simulink model "Left_Ventricular_PV_Loop_Control_2017b"  (R2017b)
settings: Solver=ode14x  StartTime=0.0  StopTime=Sim_Time  FixedStep=1/1024  MaxStep=0.01  MinStep=1E-6  RelTol=1e-5
values from neighbouring files (symbols this model uses):
  Force_Rate = 500    [Left_Ventricular_PV_Loop_Variable_Load_and_Plot.m]
  Iso_Contraction_Offset = 1    [Left_Ventricular_PV_Loop_Variable_Load_and_Plot.m]
  Resistance = 0.045    [Left_Ventricular_PV_Loop_Variable_Load_and_Plot.m]
  Systolic_Ejection_Increase = 9    [Left_Ventricular_PV_Loop_Variable_Load_and_Plot.m]
  Systolic_Ejection_Offset = [20 20]    [Left_Ventricular_PV_Loop_Variable_Load_and_Plot.m]
  Variable_Ea_C0 = [235.76 235.76 235.76 220.7 205.63 190.56 175.5 160.43]    [Left_Ventricular_PV_Loop_Variable_Load_and_Plot.m]
  Variable_Ea_C1 = [-1.4054 -1.4054 -1.4054 -1.3994 -1.3934 -1.3874 -1.3814 -1.3754]    [Left_Ventricular_PV_Loop_Variable_Load_and_Plot.m]
  Variable_EDPVR_B0 = -0.010234    [Left_Ventricular_PV_Loop_Variable_Load_and_Plot.m]
  Variable_EDPVR_B1 = 0.15836    [Left_Ventricular_PV_Loop_Variable_Load_and_Plot.m]
  Variable_EDPVR_B2 = -0.0025351    [Left_Ventricular_PV_Loop_Variable_Load_and_Plot.m]
  Variable_EDPVR_B3 = 1.4046E-5    (= 1.4046e-05)    [Left_Ventricular_PV_Loop_Variable_Load_and_Plot.m]
  Variable_ESPVR_A0 = 72.586    [Left_Ventricular_PV_Loop_Variable_Load_and_Plot.m]
  Variable_ESPVR_A1 = [0.99741 0.99741]    [Left_Ventricular_PV_Loop_Variable_Load_and_Plot.m]
libraries: fl_lib x15, nesl_utility x9, sh_lib x4, simulink x3
settings Model: SimulationMode=accelerator  Creator=ULCajunAdmin  LastModifiedBy=jmk9354
settings SolverCC: ExtrapolationOrder=2  MaxConsecutiveMinStep=5  ZeroCrossAlgorithm=Adaptive  SolverResetMethod=Robust
settings DataIOCC: SaveFormat=StructureWithTime
settings OptimizationCC: LifeSpan=inf
settings DebuggingCC: IgnoredZcDiagnostic=none  SFUnexpectedBacktrackingDiag=warning  SFNoUnconditionalDefaultTransitionDiag=warning  SFExecutionAtInitializationDiag=none
settings HardwareCC: ProdBitPerPointer=32  ProdBitPerSizeT=32  ProdBitPerPtrDiffT=32  ProdLargestAtomicFloat=None  ProdIntDivRoundTo=Undefined  ProdEndianess=Unspecified  ProdWordSize=32  ProdHWDeviceType=32-bit Generic
settings ModelReferenceCC: PropagateSignalLabelsOutOfModel=off
settings CodeAppCC: StateflowObjectComments=on
settings GRTTargetCC: TargetLangStandard=C89/C90 (ANSI)  GeneratePreprocessorConditionals=Disable all
settings ConfigComp: CovMetricSettings=dw  CovHtmlReporting=on  CovSaveCumulativeToWorkspaceVar=on  CovSaveSingleToWorkspaceVar=on  CovExternalEMLEnable=off
settings SimscapeCC: SimscapeNormalizeSystem=off

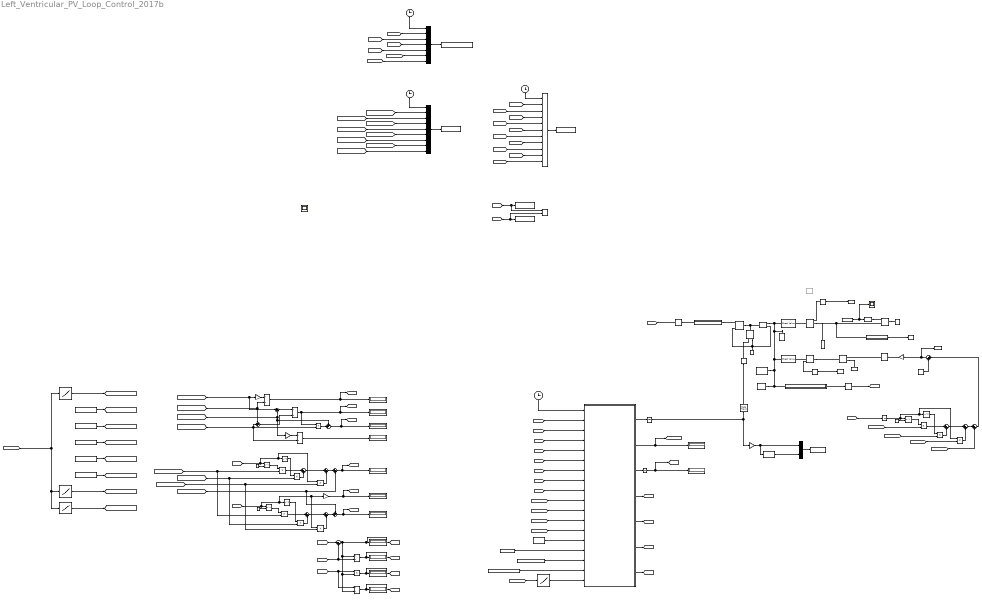
== system Left_Ventricular_PV_Loop_Control_2017b ==
   {,,,} (4 alike) : Product
  " " : Constant  Value=3
   {,,,,} (5 alike) : Product  Inputs=*/
  " " : Constant  Value=3
  " " : Constant  Value=3
  " " : Product  Inputs=**
  " " : Product  Inputs=**
  "            " : Gain  Gain=-1
  "                             " : Gain  Gain=-1
  "                                              " : Product
  "                                                              " : Product
  "                                                               " : Gain
  "                                                                        " : Product
  "                                                                            " : Product
  "                                                                            1" : Product
  Aortic Pressure Sensor : Subsystem
  Bus Creator : BusCreator  Inputs=9
  Bus Creator1 : BusCreator  Inputs=11
  Bus Creator2 : BusCreator  Inputs=2
  Bus Creator3 : BusCreator  Inputs=7
  Check Valve (Aortic Valve) Max Passage Area: 3.14*0.46^2 Cracking Pressure: 0.01 psi = 0.5 mmHg Max Opening Pressure: 0.02 psi = 1 mmHg : sh_lib/Valves/Directional Valves/Check Valve  area_max=3.14*0.46^2 in^2  pres_crack=0.01 psi  pres_max=0.02 psi  C_d=0.7  A_leak=1e-12 m^2  lam_spec=2  B_lam=0.999  Re_cr=12  dynamic=0  tau=0.001 s  area_init=1e-12 m^2
      settings: SourceProductName=Simscape Fluids  SourceProductBaseCode=SH
  "Check Valve (Mitral Valve) Max Passage Area: 3.14*0.46^2 Cracking Pressure: 0.01 psi = 0.5 mmHg Max Opening Pressure: 0.02 psi = 1 mmHg " : sh_lib/Valves/Directional Valves/Check Valve  area_max=3.14*0.46^2 in^2  pres_crack=0.01 psi  pres_max=0.02 psi  C_d=0.7  A_leak=1e-12 m^2  lam_spec=2  B_lam=0.999  Re_cr=12  dynamic=0  tau=0.001 s  area_init=1e-12 m^2
      settings: SourceProductName=Simscape Fluids  SourceProductBaseCode=SH
  Clock{,1..3} (4 alike) : Clock
  Constant Volume Hydraulic Chamber Chamber internal Diameter: 2 inch Cylindrical chamber length: 3 inch : fl_lib/Hydraulic/Hydraulic Elements/Constant Volume Hydraulic Chamber  ch_sp=2  wall_type=1  ch_volume=200 cm^3  d_in=2 in  length=3 in  pr_r_coef=1.2e-12 m/Pa  time_const=0.01 s  k_sh=1.4  pressure_specify=off  pressure_priority=High  pressure=0 Pa  pressure_nominal_specify=off  pressure_nominal_unit=Pa  pressure_nominal_value=1  diameter_incr_specify=off  diameter_incr_priority=High  diameter_incr=2 in  diameter_incr_nominal_specify=off  diameter_incr_nominal_unit=m  diameter_incr_nominal_value=1  flow_rate_specify=off  flow_rate_priority=None  flow_rate=0.001 m^3/s  flow_rate_nominal_specify=off  flow_rate_nominal_unit=m^3/s  flow_rate_nominal_value=1
      settings: SourceProductName=Simscape  SourceProductBaseCode=SS
  Cubic : Math  Operator=pow  SaturateOnIntegerOverflow=on
  "Cubic " : Math  Operator=pow  SaturateOnIntegerOverflow=on
  "Cubic " : Math  Operator=pow  SaturateOnIntegerOverflow=on
  "Discrete Derivative " : simulink/Discrete/Discrete Derivative  gainval=1.0  ICPrevScaledInput=0.0  OutMin=[]  OutMax=[]  OutDataType=fixdt(1, 16)  OutScaling=2^-10  DoSatur=off
  "EDPVR - B0 " : Constant  Value=Variable_EDPVR_B0  SampleTime=1/1024
  "EDPVR - B1 " : Constant  Value=Variable_EDPVR_B1  SampleTime=1/1024
  "EDPVR - B2 " : Constant  Value=Variable_EDPVR_B2  SampleTime=1/1024
  "EDPVR - B3 " : Constant  Value=Variable_EDPVR_B3  SampleTime=1/1024
  "ESPVR - A0 " : Constant  Value=Variable_ESPVR_A0  SampleTime=1/1024
  ESPVR - A1 1-D Lookup Table : Lookup_n-D  NumberOfTableDimensions=1  BreakpointsSpecification=Even spacing  BreakpointsForDimension1=[-5:5]  Table=Variable_ESPVR_A1  InterpMethod=Nearest  ExtrapMethod=Clip  UseLastTableValue=on  InternalRulePriority=Speed  RndMeth=Simplest  InputSameDT=on
  Ea - C0 1-D Lookup Table : Lookup_n-D  NumberOfTableDimensions=1  BreakpointsSpecification=Even spacing  BreakpointsForDimension1=[-5:5]  Table=Variable_Ea_C0  InterpMethod=Nearest  ExtrapMethod=Clip  UseLastTableValue=on  InternalRulePriority=Speed  RndMeth=Simplest  InputSameDT=on
  Ea - C1 1-D Lookup Table : Lookup_n-D  NumberOfTableDimensions=1  BreakpointsSpecification=Even spacing  BreakpointsForDimension1=[-5:5]  Table=Variable_Ea_C1  InterpMethod=Nearest  ExtrapMethod=Clip  UseLastTableValue=on  InternalRulePriority=Speed  RndMeth=Simplest  InputSameDT=on
  Force Rate : Constant  Value=Force_Rate  SampleTime=1/1024
  Gain2 : Gain  Gain=-1
  Heart Beat Cycle Number : Display
  Heart Rate : Display
  Hydraulic Flow Rate Sensor : fl_lib/Hydraulic/Hydraulic Sensors/Hydraulic Flow Rate Sensor
      settings: SourceProductName=Simscape
  "Hydraulic Flow Rate Sensor " : fl_lib/Hydraulic/Hydraulic Sensors/Hydraulic Flow Rate Sensor
      settings: SourceProductName=Simscape
  Hydraulic Fluid Glycerol/Water Mixture : fl_lib/Hydraulic/Hydraulic Utilities/Custom Hydraulic Fluid  density=1107.1 kg/m^3  viscosity_kin=3.3 cSt  bulk=0.8e9 Pa  alpha=0.005  range_error=2
      settings: SourceProductName=Simscape  SourceProductBaseCode=SS
  "Hydraulic Pressure Source " : fl_lib/Hydraulic/Hydraulic Sources/Hydraulic Pressure Source
      settings: SourceProductName=Simscape  SourceProductBaseCode=SS
  "Hydraulic Reference " : fl_lib/Hydraulic/Hydraulic Elements/Hydraulic Reference
      settings: SourceProductName=Simscape
  "Hydraulic Reference   " : fl_lib/Hydraulic/Hydraulic Elements/Hydraulic Reference
      settings: SourceProductName=Simscape
  "Ideal Force Source " : fl_lib/Mechanical/Mechanical Sources/Ideal Force Source
  "Ideal Translational Motion Sensor Initial Position: 0 inch " : fl_lib/Mechanical/Mechanical Sensors/Ideal Translational Motion Sensor  offset=0 in
  Isovolumetric Contraction Offset : Constant  Value=Iso_Contraction_Offset  SampleTime=1/1024
  LAP [mmHg] Offset : Constant  Value=2
  Left Ventricle Pressure Sensor : Subsystem
  Left Ventricular Arterial Elastance [mmHg/mL] : Display
  Left Ventricular Ejection Fraction : Display
  Left Ventricular End-Diastolic Pressure [mmHg] : Display
  Left Ventricular End-Diastolic Volume [mL] : Display
  Left Ventricular End-Isovolumetric Relaxation Pressure [mmHg] : Display
  Left Ventricular End-Isovolumetric Relaxation Volume [mL] : Display
  Left Ventricular End-Systolic Pressure [mmHg] : Display
  Left Ventricular End-Systolic Volume [mL] : Display
  Left Ventricular Stroke Volume [mL] : Display
  Left Ventricular Stroke Work [mmHg*mL] : Display
  Left Ventricular Volume Conversion : Subsystem
  Mechanical Translational Reference : fl_lib/Mechanical/Translational Elements/Mechanical Translational Reference
  "Needle Valve Orifice Diameter: 0.5 inch Needle Cone Angle: 90 degrees " : sh_lib/Valves/Flow Control Valves/Needle Valve  d_orif=0.5 in  cone_angle=90 deg  x_0=0 in  C_d=0.65  A_leak=1e-12 m^2  lam_spec=2  B_lam=0.999  Re_cr=10
      settings: SourceProductName=Simscape Fluids  SourceProductBaseCode=SH
  Needle Valve Resistance: Variable : Constant  Value=Resistance  VectorParams1D=off
  PS-Simulink Converter (mL/min) : nesl_utility/PS-Simulink Converter  PhysicalDomain=network_engine_domain  SubClassName=ps_output  LeftPortType=input  RightPortType=output  PseudoPeriodic=off  Frequencies=[]  Unit=cm^3/min  AffineConversion=off
  "PS-Simulink Converter (mL/min) " : nesl_utility/PS-Simulink Converter  PhysicalDomain=network_engine_domain  SubClassName=ps_output  LeftPortType=input  RightPortType=output  PseudoPeriodic=off  Frequencies=[]  Unit=cm^3/min  AffineConversion=off
  Piston Cross-Sectional Area : Constant  Value=pi*2.54^2  SampleTime=1/1024
  Ramp : simulink/Sources/Ramp  Commented=on  slope=0.0125  start=2  X0=0
  Rate Transition 512 Hz : RateTransition  OutPortSampleTime=1/512
  Rate Transition to 512 Hz : RateTransition  OutPortSampleTime=1/512
  "Rate Transition to 512 Hz " : RateTransition  OutPortSampleTime=1/512
  Scope3 : Scope
  "Simulink-PS Converter (Newtons) " : nesl_utility/Simulink-PS Converter  PhysicalDomain=network_engine_domain  SubClassName=ps_input  LeftPortType=input  RightPortType=output  PseudoPeriodic=off  Frequencies=[]  NoiseDistribution=none  NoiseParameters=[]  Unit=N  AffineConversion=off  FilteringAndDerivatives=filter  SimscapeFilterOrder=1  InputFilterTimeConstant=.005  UdotUserProvided=1
  Simulink-PS Converter (inch) : nesl_utility/Simulink-PS Converter  PhysicalDomain=network_engine_domain  SubClassName=ps_input  LeftPortType=input  RightPortType=output  PseudoPeriodic=off  Frequencies=[]  NoiseDistribution=none  NoiseParameters=[]  Unit=in  AffineConversion=off  FilteringAndDerivatives=filter  SimscapeFilterOrder=1  InputFilterTimeConstant=0.001  UdotUserProvided=1
  "Simulink-PS Converter (psi) " : nesl_utility/Simulink-PS Converter  PhysicalDomain=network_engine_domain  SubClassName=ps_input  LeftPortType=input  RightPortType=output  PseudoPeriodic=off  Frequencies=[]  NoiseDistribution=none  NoiseParameters=[]  Unit=psi  AffineConversion=off  FilteringAndDerivatives=filter  SimscapeFilterOrder=1  InputFilterTimeConstant=.005  UdotUserProvided=1
  "Solver Configuration " : nesl_utility/Solver Configuration  PhysicalDomain=network_engine_domain  SubClassName=solver  LeftPortType=input  RightPortType=generic  Tones=[]  Harmonics=[]  SimulateNoise=off  Profile=off  UseLocalSampling=off  EnableSwitchedLinearOptims=on  FrequencyDomain=off  UseCCode=off  RelTol=0.001  AbsTol=1e-06  MinStep=1e-09  ToWorkspace=off  RevertToSquareIcSolve=off  NumHomotopyIterations=100  PhasorMode=off  PhasorModeNumHarmonics=1  DoDC=off  ResidualTolerance=1e-09  UseLocalSolver=on  LocalSolverChoice=NE_BACKWARD_EULER_ADVANCER  LocalSolverSampleTime=1/1024  DoFixedCost=on  MaxNonlinIter=3  MaxModeIter=2  LinearAlgebra=Sparse  EquationFormulation=NE_TIME_EF  DelaysMemoryBudget=1024  AutomaticFiltering=on  FilteringTimeConstant=0.001
  Spring-Loaded Accumulator Fluid Chamber Capacity: 517.15 mL Preload Pressure (gauge): Variable psi Pressure at Full Capacity (gauge): Variable psi Initial Volume of Fluid: Variable mL : sh_lib/Accumulators/Spring-Loaded Accumulator  capacity=Fluid_Chamber_Capacity cm^3  pr_preload=Preload_Pressure psi  pr_max=Pressure_Full_Capacity psi  stiff_coeff=1e10 Pa/m^3  penetr_coeff=1e10 s*Pa/m^6  flow_rate_specify=off  flow_rate_priority=None  flow_rate=0.005 m^3/s  flow_rate_nominal_specify=off  flow_rate_nominal_unit=m^3/s  flow_rate_nominal_value=1  fluid_volume_specify=on  fluid_volume_priority=High  fluid_volume=Volume_of_Fluid cm^3  fluid_volume_nominal_specify=off  fluid_volume_nominal_unit=m^3  fluid_volume_nominal_value=1  fluid_pressure_specify=off  fluid_pressure_priority=None  fluid_pressure=1.01325e+5 Pa  fluid_pressure_nominal_specify=off  fluid_pressure_nominal_unit=Pa  fluid_pressure_nominal_value=1
      settings: SourceProductName=Simscape Fluids  SourceProductBaseCode=SH
  Square : Math  Operator=square  SaturateOnIntegerOverflow=on
  "Square " : Math  Operator=square  SaturateOnIntegerOverflow=on
  Square1 : Math  Operator=square  SaturateOnIntegerOverflow=on
  State Transition Table : State Transition Table  TreatAsAtomicUnit=on
  Sum : Sum  Inputs=|+-
  Sum1 : Sum  Inputs=-+|
  Sum{3..5,7..8,11..14} (9 alike) : Sum  Inputs=|++
  Sum2 : Sum  Inputs=++|
  Sum6 : Sum  Inputs=|-+
  Sum9 : Sum  Inputs=++|
  Systolic Ejection Decrease : Constant  Value=Systolic_Ejection_Increase  SampleTime=1/1024
  Systolic Ejection Offset 1-D Lookup Table : Lookup_n-D  NumberOfTableDimensions=1  BreakpointsSpecification=Even spacing  BreakpointsForDimension1=[-5:5]  Table=Systolic_Ejection_Offset  InterpMethod=Nearest  ExtrapMethod=Clip  UseLastTableValue=on  InternalRulePriority=Speed  RndMeth=Simplest  InputSameDT=on
  To Workspace : ToWorkspace  VariableName=Measured_LVV  SaveFormat=Structure With Time  SampleTime=1/1024
  To Workspace Aortic Pressure [mmHg] : ToWorkspace  VariableName=AoP  SaveFormat=Structure With Time  SampleTime=1/1024
  To Workspace Computational Values : ToWorkspace  VariableName=Computational_Values  SaveFormat=Structure With Time  SampleTime=1/1024
  To Workspace Contraint Constants : ToWorkspace  VariableName=Constraint_Constants  SaveFormat=Structure With Time  SampleTime=1/1024
  To Workspace Drive Signal : ToWorkspace  VariableName=Drive_Signal  SaveFormat=Structure With Time  SampleTime=1/1024
  To Workspace Left Atrial Pressure [mmHg] : ToWorkspace  VariableName=LAP  SaveFormat=Structure With Time  SampleTime=1/1024
  To Workspace Left Ventricular Inflow [mL/min] : ToWorkspace  VariableName=LVIF  SaveFormat=Structure With Time  SampleTime=1/1024
  To Workspace Left Ventricular Outflow [mL/min] : ToWorkspace  VariableName=LVOF  SaveFormat=Structure With Time  SampleTime=1/1024
  "To Workspace Phase Change, Heart Beat Cycle Count, and Heart Rate" : ToWorkspace  VariableName=PhaseChange_HeartBeatCount_HeartRate  SaveFormat=Structure With Time  SampleTime=1/1024
  To Workspace2 : ToWorkspace  VariableName=Measured_LVP  SaveFormat=Structure With Time  SampleTime=1/1024
  Translational Hydro-Mechanical Converter Piston Area: pi*2.54^2 cm^2 Converter Orientation: Positive Direction : fl_lib/Hydraulic/Hydraulic Elements/Translational Hydro-Mechanical Converter  area=3.14*1^2 in^2  or=1  compressibility=0  init_pos=0 m  V_dead=1e-4 m^3  k_sh=1.4  initial_pressure=0 Pa
      settings: SourceProductName=Simscape  SourceProductBaseCode=SS
  "Unit Converter: mmHg to psi " : Gain  Gain=1/51.715
  Unit Delay to Prevent Algebraic Loop : UnitDelay  InitialCondition=1  SampleTime=-1
  "Unit Delay to Prevent Algebraic Loop " : UnitDelay  InitialCondition=1  SampleTime=-1
  "Unit Delay to Prevent Algebraic Loop  " : UnitDelay  InitialCondition=1  SampleTime=-1
  Vo [mL] : Display
  XY Graph : simulink/Sinks/XY Graph  xmin=-50  xmax=300  ymin=-50  ymax=300  st=-1
  Scope : Scope
  wires:
  Left Ventricle Pressure Sensor/1(Pressure Gauge [mmHg]) -> "Rate Transition to 512 Hz "/1  "LVP"
  Left Ventricular Volume Conversion/1(Vol [mL]) -> Rate Transition to 512 Hz/1  "LVV [mL]"
  Clock/1 -> State Transition Table/1(Time)  "Time"
  Needle Valve Resistance: Variable/1 -> Scope3/1, Simulink-PS Converter (inch)/1
  [LVV] -> XY Graph/1, To Workspace/1  "LVV [mL]"
  Aortic Pressure Sensor/1(Pgauge [mmHg]) -> To Workspace Aortic Pressure [mmHg]/1  "AoP [mmHg]"
  [LVP] -> XY Graph/2, To Workspace2/1  "LVP [mmHg]"
  "Discrete Derivative "/1 -> Bus Creator2/2  "Derivative of Drive Signal"
  Gain2/1 -> Bus Creator2/1, "Discrete Derivative "/1  "Drive Signal - Force [N]"
  Square/1 -> "                                                                            "/1
  [EDPVR_B2] -> "                                                              "/2, "                                                                            "/2  "B2"
  " "/1 -> [LVef], Left Ventricular Ejection Fraction/1  "LVef"
  Sum2/1 -> Left Ventricular End-Systolic Pressure [mmHg]/1, [LVesp]  "LVesp"
  Sum4/1 -> Sum5/1
  "                                                                        "/1 -> Sum4/2
  " "/1 -> [LVea], Left Ventricular Arterial Elastance [mmHg/mL]/1  "LVea"
  [EDPVR_B3] -> " "/2, "                                              "/2  "B3"
  "Square "/1 -> "                                                              "/1
  [ESPVR_A1] -> " "/2, Sum1/2, " "/2  "A1"
  " "/1 -> Sum7/1
  [Ea_C1] -> " "/2, Sum1/1  "C1"
  [EDPVR_B1] -> "                                                                        "/2, " "/2  "B1"
  " "/1 -> Sum2/2
  "                                                               "/1 -> [LVeirv], Left Ventricular End-Isovolumetric Relaxation Volume [mL]/1  "LVeirv"
  Sum6/1 -> [LVsv], Left Ventricular Stroke Volume [mL]/1, " "/2, " "/2, " "/1  "LVsv"
  [LVesv] -> Sum6/1  "LVesv"
  Sum/1 -> " "/1  "(C0-A0)"
  "                                                              "/1 -> Sum3/2
  Sum9/1 -> [LVeirp], Left Ventricular End-Isovolumetric Relaxation Pressure [mmHg]/1  "LVeirp"
  "                                              "/1 -> Sum3/1
  "Cubic "/1 -> " "/1
  [LVesv] -> "                                                               "/1, " "/1, Square/1, "Cubic "/1  "LVesv"
  Sum3/1 -> Sum4/1
  [Ea_C0] -> "            "/1, Sum/1  "C0"
  [LVedv] -> "                                                                        "/1, "Square "/1, Cubic/1  "LVedv"
  [ESPVR_A0] -> Sum/2, "                             "/1, Sum2/1  "A0"
  Sum8/1 -> Sum9/2
  [EDPVR_B0] -> Sum9/1, Sum5/2  "B0"
  Sum1/1 -> " "/2  "(A1-C1)"
  " "/1 -> Left Ventricular End-Diastolic Volume [mL]/1, [LVedv]  "LVedv"
  [LVedv] -> Sum6/2, " "/2  "LVedv"
  " "/1 -> [LVsw], Left Ventricular Stroke Work [mmHg*mL]/1  "LVsw"
  " "/1 -> Cubic/2
  " "/1 -> Vo [mL]/1
  [LVesp] -> " "/1, " "/1  "LVesp"
  "                                                                            "/1 -> Sum7/2
  Sum7/1 -> Sum8/1
  Sum5/1 -> Left Ventricular End-Diastolic Pressure [mmHg]/1, [LVedp]  "LVedp"
  "                             "/1 -> " "/1
  "            "/1 -> " "/1
  " "/1 -> " "/1, [LVesv], Left Ventricular End-Systolic Volume [mL]/1  "LVesv"
  " "/1 -> Sum8/2
  " "/1 -> "Cubic "/2
  Cubic/1 -> "                                              "/1
  [LVP] -> State Transition Table/2(Pressure)  "Measured LVP [mmHg]"
  [LVV] -> State Transition Table/3(Volume)  "Measured LVV [mL]"
  [LVesv] -> State Transition Table/5(LVesv)  "LVesv"
  [LVedv] -> State Transition Table/7(LVedv)  "LVedv"
  [LVesp] -> State Transition Table/4(LVesp)  "LVesp"
  [LVedp] -> State Transition Table/6(LVedp)  "LVedp"
  [LVeirp] -> State Transition Table/8(LVeirp)  "LVeirp"
  [LVeirv] -> State Transition Table/9(LVeirv)  "LVeirv"
  State Transition Table/1(Force) -> Unit Delay to Prevent Algebraic Loop/1
  [EDPVR_B3] -> State Transition Table/10(b3)  "b3"
  [EDPVR_B2] -> State Transition Table/11(b2)  "b2"
  [EDPVR_B1] -> State Transition Table/12(b1)  "b1"
  [EDPVR_B0] -> State Transition Table/13(b0)  "b0"
  Piston Cross-Sectional Area/1 -> State Transition Table/14(Piston_Area)  "Piston Area"
  Unit Delay to Prevent Algebraic Loop/1 -> Gain2/1, Rate Transition 512 Hz/1
  Bus Creator/1 -> To Workspace Contraint Constants/1
  [EDPVR_B0] -> Bus Creator/7  "EDPVR_B0"
  [EDPVR_B1] -> Bus Creator/6  "EDPVR_B1"
  [EDPVR_B2] -> Bus Creator/5  "EDPVR_B2"
  [EDPVR_B3] -> Bus Creator/4  "EDPVR_B3"
  [Ea_C0] -> Bus Creator/9  "Ea_C0_Preload"
  [Ea_C1] -> Bus Creator/8  "Ea_C1_Afterload"
  [ESPVR_A1] -> Bus Creator/2  "ESPVR_A1_Contractility"
  [ESPVR_A0] -> Bus Creator/3  "ESPVR_A0"
  Bus Creator1/1 -> To Workspace Computational Values/1
  [LVesp] -> Bus Creator1/2  "LVesp [mmHg]"
  [LVesv] -> Bus Creator1/3  "LVesv [mL]"
  [LVedp] -> Bus Creator1/4  "LVedp [mmHg]"
  [LVedv] -> Bus Creator1/5  "LVedv [mL]"
  [LVeirp] -> Bus Creator1/6  "LVeirp [mmHg]"
  [LVeirv] -> Bus Creator1/7  "LVeirv [mL]"
  [LVsv] -> Bus Creator1/8  "LVsv [mL]"
  [LVea] -> Bus Creator1/11  "LVea [mmHg/mL]"
  [LVsw] -> Bus Creator1/10  "LVsw [mmHg*mL]"
  [LVef] -> Bus Creator1/9  "LVef"
  Bus Creator2/1 -> To Workspace Drive Signal/1
  State Transition Table/2(HeartRate) -> [Heart_Rate], Heart Rate/1
  Rate Transition 512 Hz/1 -> "Simulink-PS Converter (Newtons) "/1
  "Unit Converter: mmHg to psi "/1 -> "Simulink-PS Converter (psi) "/1
  Sum11/1 -> To Workspace Left Atrial Pressure [mmHg]/1, "Unit Converter: mmHg to psi "/1  "LAP [mmHg]"
  LAP [mmHg] Offset/1 -> Sum11/2
  "                                                                            1"/1 -> Sum12/2
  "Cubic "/1 -> " "/1
  " "/1 -> Sum13/2
  [EDPVR_B0] -> Sum14/2  "B0"
  Sum12/1 -> Sum13/1
  [LVV] -> "Unit Delay to Prevent Algebraic Loop "/1  "Measured LVV [mL]"
  " "/1 -> Sum12/1
  " "/1 -> "Cubic "/2
  Sum13/1 -> Sum14/1
  Square1/1 -> "                                                                            1"/1
  [EDPVR_B3] -> " "/2  "B3"
  [EDPVR_B2] -> "                                                                            1"/2  "B2"
  [EDPVR_B1] -> " "/2  "B1"
  Sum14/1 -> Sum11/1
  Clock1/1 -> Bus Creator/1  "Time"
  Clock2/1 -> Bus Creator1/1  "Time"
  State Transition Table/3(Count) -> "Unit Delay to Prevent Algebraic Loop  "/1
  "Unit Delay to Prevent Algebraic Loop  "/1 -> Heart Beat Cycle Number/1, [Count]
  State Transition Table/4(Phase_1) -> [Phase_1]
  State Transition Table/5(Phase_2) -> [Phase_2]
  State Transition Table/6(Phase_3) -> [Phase_3]
  State Transition Table/7(Phase_4) -> [Phase_4]
  Bus Creator3/1 -> "To Workspace Phase Change, Heart Beat Cycle Count, and Heart Rate"/1
  Clock3/1 -> Bus Creator3/1  "Time"
  [Phase_1] -> Bus Creator3/2  "Phase 1"
  [Phase_2] -> Bus Creator3/3  "Phase 2"
  [Phase_3] -> Bus Creator3/4  "Phase 3"
  [Phase_4] -> Bus Creator3/5  "Phase 4"
  [Count] -> Ea - C0 1-D Lookup Table/1, Ea - C1 1-D Lookup Table/1, ESPVR - A1 1-D Lookup Table/1  "Heartbeat Cycle Count"
  "Unit Delay to Prevent Algebraic Loop "/1 -> " "/1, Square1/1, "Cubic "/1
  "ESPVR - A0 "/1 -> [ESPVR_A0]
  ESPVR - A1 1-D Lookup Table/1 -> [ESPVR_A1]
  "EDPVR - B3 "/1 -> [EDPVR_B3]
  "EDPVR - B0 "/1 -> [EDPVR_B0]
  "EDPVR - B1 "/1 -> [EDPVR_B1]
  "EDPVR - B2 "/1 -> [EDPVR_B2]
  Ea - C0 1-D Lookup Table/1 -> [Ea_C0]
  Ea - C1 1-D Lookup Table/1 -> [Ea_C1]
  [Count] -> Bus Creator3/6  "Heartbeat Cycle Count"
  [Heart_Rate] -> Bus Creator3/7  "Heart Rate"
  PS-Simulink Converter (mL/min)/1 -> To Workspace Left Ventricular Outflow [mL/min]/1  "LVOF [mL/min]"
  Force Rate/1 -> State Transition Table/15(Force_Rate)  "Force Rate"
  Isovolumetric Contraction Offset/1 -> State Transition Table/16(Iso_Contraction_Offset)  "Isovolumetric Contraction Offset"
  Systolic Ejection Decrease/1 -> State Transition Table/17(Systolic_Ejection_Increase)  "Systolic Ejection Increase"
  Systolic Ejection Offset 1-D Lookup Table/1 -> State Transition Table/18(Systolic_Ejection_Offset)  "Systolic Ejection Offset"
  [Count] -> Systolic Ejection Offset 1-D Lookup Table/1
  "PS-Simulink Converter (mL/min) "/1 -> To Workspace Left Ventricular Inflow [mL/min]/1  "LVIF [mL/min]"
  Rate Transition to 512 Hz/1 -> [LVV]  "LVV [mL]"
  "Rate Transition to 512 Hz "/1 -> [LVP]  "LVP [mmHg]"
  connections:
  Mechanical Translational Reference/LConn1 -- Translational Hydro-Mechanical Converter Piston Area: pi*2.54^2 cm^2 Converter Orientation: Positive Direction/LConn1 -- "Ideal Force Source "/RConn2 -- "Ideal Translational Motion Sensor Initial Position: 0 inch "/RConn1
  Aortic Pressure Sensor/LConn1 -- "Hydraulic Flow Rate Sensor "/RConn2 -- Spring-Loaded Accumulator Fluid Chamber Capacity: 517.15 mL Preload Pressure (gauge): Variable psi Pressure at Full Capacity (gauge): Variable psi Initial Volume of Fluid: Variable mL/RConn1 -- "Needle Valve Orifice Diameter: 0.5 inch Needle Cone Angle: 90 degrees "/LConn2
  "Ideal Translational Motion Sensor Initial Position: 0 inch "/LConn1 -- "Ideal Force Source "/LConn1 -- Translational Hydro-Mechanical Converter Piston Area: pi*2.54^2 cm^2 Converter Orientation: Positive Direction/RConn1
  "Hydraulic Pressure Source "/RConn2 -- "Hydraulic Reference   "/LConn1
  "Needle Valve Orifice Diameter: 0.5 inch Needle Cone Angle: 90 degrees "/RConn1 -- "Hydraulic Reference "/LConn1
  Left Ventricular Volume Conversion/LConn1 -- "Ideal Translational Motion Sensor Initial Position: 0 inch "/RConn3
  Simulink-PS Converter (inch)/RConn1 -- "Needle Valve Orifice Diameter: 0.5 inch Needle Cone Angle: 90 degrees "/LConn1
  Hydraulic Flow Rate Sensor/RConn2 -- "Check Valve (Mitral Valve) Max Passage Area: 3.14*0.46^2 Cracking Pressure: 0.01 psi = 0.5 mmHg Max Opening Pressure: 0.02 psi = 1 mmHg "/LConn1
  Left Ventricle Pressure Sensor/LConn1 -- Constant Volume Hydraulic Chamber Chamber internal Diameter: 2 inch Cylindrical chamber length: 3 inch/LConn1 -- Translational Hydro-Mechanical Converter Piston Area: pi*2.54^2 cm^2 Converter Orientation: Positive Direction/LConn2 -- Check Valve (Aortic Valve) Max Passage Area: 3.14*0.46^2 Cracking Pressure: 0.01 psi = 0.5 mmHg Max Opening Pressure: 0.02 psi = 1 mmHg/LConn1 -- "Check Valve (Mitral Valve) Max Passage Area: 3.14*0.46^2 Cracking Pressure: 0.01 psi = 0.5 mmHg Max Opening Pressure: 0.02 psi = 1 mmHg "/RConn1 -- Hydraulic Fluid Glycerol/Water Mixture/RConn1 -- "Solver Configuration "/RConn1
  "Simulink-PS Converter (Newtons) "/RConn1 -- "Ideal Force Source "/RConn1
  "Simulink-PS Converter (psi) "/RConn1 -- "Hydraulic Pressure Source "/RConn1
  "Hydraulic Flow Rate Sensor "/LConn1 -- Check Valve (Aortic Valve) Max Passage Area: 3.14*0.46^2 Cracking Pressure: 0.01 psi = 0.5 mmHg Max Opening Pressure: 0.02 psi = 1 mmHg/RConn1
  "Hydraulic Flow Rate Sensor "/RConn1 -- PS-Simulink Converter (mL/min)/LConn1
  Hydraulic Flow Rate Sensor/LConn1 -- "Hydraulic Pressure Source "/LConn1
  Hydraulic Flow Rate Sensor/RConn1 -- "PS-Simulink Converter (mL/min) "/LConn1

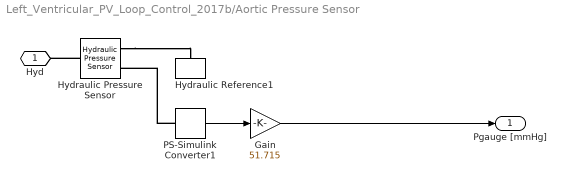
== system Left_Ventricular_PV_Loop_Control_2017b/Aortic Pressure Sensor ==
  Gain : Gain  Gain=51.715
  Hydraulic Pressure Sensor : fl_lib/Hydraulic/Hydraulic Sensors/Hydraulic Pressure Sensor
      settings: SourceProductName=Simscape
  Hydraulic Reference1 : fl_lib/Hydraulic/Hydraulic Elements/Hydraulic Reference
      settings: SourceProductName=Simscape
  PS-Simulink Converter1 : nesl_utility/PS-Simulink Converter  PhysicalDomain=network_engine_domain  SubClassName=ps_output  LeftPortType=input  RightPortType=output  PseudoPeriodic=off  Frequencies=[]  Unit=psi  AffineConversion=off
  Hyd : PMIOPort  Side=Left
  Pgauge [mmHg] : Outport
  wires:
  PS-Simulink Converter1/1 -> Gain/1
  Gain/1 -> Pgauge [mmHg]/1
  connections:
  PS-Simulink Converter1/LConn1 -- Hydraulic Pressure Sensor/RConn2
  Hydraulic Pressure Sensor/RConn1 -- Hydraulic Reference1/LConn1
  Hydraulic Pressure Sensor/LConn1 -- Hyd/RConn1

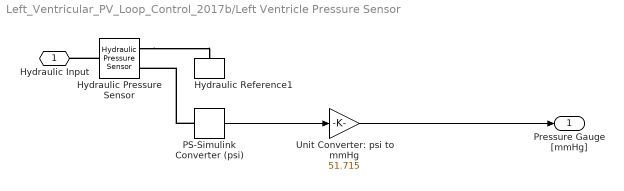
== system Left_Ventricular_PV_Loop_Control_2017b/Left Ventricle Pressure Sensor ==
  "Hydraulic Pressure Sensor " : fl_lib/Hydraulic/Hydraulic Sensors/Hydraulic Pressure Sensor
      settings: SourceProductName=Simscape
  Hydraulic Reference1 : fl_lib/Hydraulic/Hydraulic Elements/Hydraulic Reference
      settings: SourceProductName=Simscape
  PS-Simulink Converter (psi) : nesl_utility/PS-Simulink Converter  PhysicalDomain=network_engine_domain  SubClassName=ps_output  LeftPortType=input  RightPortType=output  PseudoPeriodic=off  Frequencies=[]  Unit=psi  AffineConversion=off
  Unit Converter: psi to mmHg : Gain  Gain=51.715
  Hydraulic Input : PMIOPort  Side=Left
  Pressure Gauge [mmHg] : Outport
  wires:
  PS-Simulink Converter (psi)/1 -> Unit Converter: psi to mmHg/1
  Unit Converter: psi to mmHg/1 -> Pressure Gauge [mmHg]/1
  connections:
  PS-Simulink Converter (psi)/LConn1 -- "Hydraulic Pressure Sensor "/RConn2
  "Hydraulic Pressure Sensor "/RConn1 -- Hydraulic Reference1/LConn1
  "Hydraulic Pressure Sensor "/LConn1 -- Hydraulic Input/RConn1

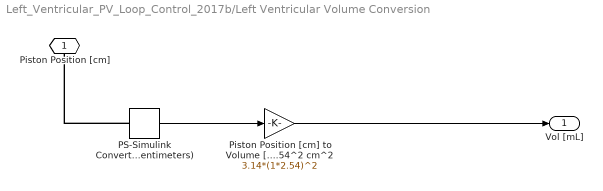
== system Left_Ventricular_PV_Loop_Control_2017b/Left Ventricular Volume Conversion ==
  PS-Simulink Converter (Centimeters) : nesl_utility/PS-Simulink Converter  PhysicalDomain=network_engine_domain  SubClassName=ps_output  LeftPortType=input  RightPortType=output  PseudoPeriodic=off  Frequencies=[]  Unit=cm  AffineConversion=off
  Piston Position [cm] to Volume [mL] Cross-Sectional Area of Piston = pi*2.54^2 cm^2 : Gain  Gain=3.14*(1*2.54)^2
  Piston Position [cm] : PMIOPort  Side=Left
  Vol [mL] : Outport
  wires:
  PS-Simulink Converter (Centimeters)/1 -> Piston Position [cm] to Volume [mL] Cross-Sectional Area of Piston = pi*2.54^2 cm^2/1
  Piston Position [cm] to Volume [mL] Cross-Sectional Area of Piston = pi*2.54^2 cm^2/1 -> Vol [mL]/1
  connections:
  PS-Simulink Converter (Centimeters)/LConn1 -- Piston Position [cm]/RConn1

== stateflow chart Left_Ventricular_PV_Loop_Control_2017b/State Transition Table ==
  settings: updateMethod=DISCRETE  sampleTime=1/1024
  state Initial
    entry:
    Force = 0;
    Count = 0;
    Phase_1 = 0;
    Phase_2 = 0;
    Phase_3 = 0;
    Phase_4 = 0;
    ED_Time = 0;
    ES_Time = 0;
    Cycle_Time = 0;
  state Info
    entry:
    HeartRate = 60/(Time - Cycle_Time);
    Count = Count + 1;
    Phase_1 = 0;
    Phase_2 = 0;
    Phase_3 = 0;
    Phase_4 = 0;
  state Diastolic_Filling % Phase 1
    entry:
    Phase_1 = 1;
    Phase_2 = 0;
    Phase_3 = 0;
    Phase_4 = 0;
  state Isovolumetric_Contraction % Phase 2
    entry:
    Phase_1 = 0;
    Phase_2 = 1;
    Phase_3 = 0;
    Phase_4 = 0;
  state Systolic_Ejection % Phase 3
    entry:
    Phase_1 = 0;
    Phase_2 = 0;
    Phase_3 = 1;
    Phase_4 = 0;
  state Isovolumetric_Relaxation % Phase 4
    entry:
    Phase_1 = 0;
    Phase_2 = 0;
    Phase_3 = 0;
    Phase_4 = 1;
  (default) -> Initial
  Initial -> Info : [after(1/1024,sec)]
  (junction 142) -> Info
  (junction 144) -> (junction 142)
  Info -> Diastolic_Filling % Phase 1 : [after(1/1024,sec)]
      | {Cycle_Time = Time;}
  Diastolic_Filling % Phase 1 -> (junction 111) [order 2] : [Volume < LVedv]
      | {Force = -1*(b3*Volume^3+b2*Volume^2+b1*Volume+b0)*(1/75.00615)*Piston_Area;}
  (junction 111) -> Diastolic_Filling % Phase 1
  Diastolic_Filling % Phase 1 -> Isovolumetric_Contraction % Phase 2 [order 1] : [Volume >= LVedv - Iso_Contraction_Offset]
      | {ED_Time = Time;}
  Isovolumetric_Contraction % Phase 2 -> (junction 87) [order 2] : [Pressure < LVesp]
      | {Force = Force - Force_Rate*(1/1024);}
  (junction 87) -> Isovolumetric_Contraction % Phase 2
  Isovolumetric_Contraction % Phase 2 -> Systolic_Ejection % Phase 3 [order 1] : [Pressure >= LVesp - Systolic_Ejection_Offset]
  Systolic_Ejection % Phase 3 -> (junction 90) [order 2] : [Volume > LVesv]
      | {Force = Force - Systolic_Ejection_Increase*(1/1024);}
  (junction 90) -> Systolic_Ejection % Phase 3
  Systolic_Ejection % Phase 3 -> Isovolumetric_Relaxation % Phase 4 [order 1] : [Volume <= LVesv+0.5]
      | {ES_Time = Time;}
  Isovolumetric_Relaxation % Phase 4 -> (junction 93) [order 2] : [Pressure > LVeirp]
      | {Force = Force + (Force_Rate/3)*(1/1024);}
  (junction 93) -> Isovolumetric_Relaxation % Phase 4
  Isovolumetric_Relaxation % Phase 4 -> (junction 144) [order 1] : [Pressure <= LVeirp]
  data: Time input; Force output; Pressure input; Volume input; LVesp input; LVesv input; LVedp input; LVedv input; LVeirp input; LVeirv input; b3 input; b2 input; b1 input; b0 input; Piston_Area input; Force_Rate input; Iso_Contraction_Offset input; HeartRate output; ED_Time local; ES_Time local; Count output; Phase_1 output; Phase_2 output; Phase_3 output; Phase_4 output; Systolic_Ejection_Increase input; Systolic_Ejection_Offset input; Cycle_Time local
